simulink model "dbm_2020b"  (R2020b)
settings: Solver=FixedStepAuto  StartTime=0.0  StopTime=50  FixedStep=0.01  RelTol=1e-3
libraries: simulink x1
settings Model: Creator=felix  LastModifiedBy=felix
settings OptimizationCC: DefaultParameterBehavior=Inlined  UseDivisionForNetSlopeComputation=on  GainParamInheritBuiltInType=on  UseFloatMulNetSlope=on  InlineInvariantSignals=on  EfficientFloat2IntCast=on  LifeSpan=1
settings DebuggingCC: SFMachineParentedDataDiag=error
settings HardwareCC: ProdLongLongMode=on
settings SFSimCC: MATLABDynamicMemAlloc=off
settings RTWCC: GenerateReport=on  LaunchReport=on
settings CodeAppCC: ForceParamTrailComments=on
settings GRTTargetCC: CombineSignalStateStructs=on  MatFileLogging=off  SupportVariableSizeSignals=on

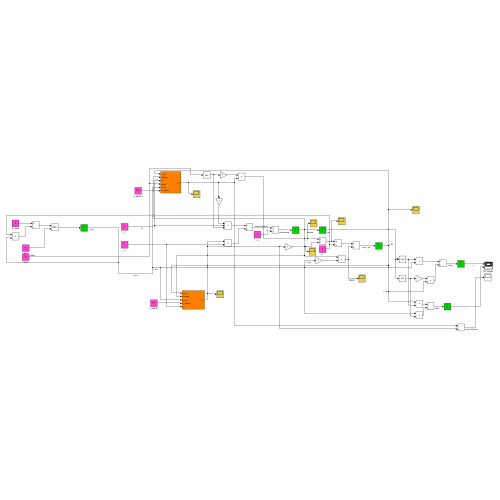
[thumbnail: Simulink's stored preview of the top-level diagram]
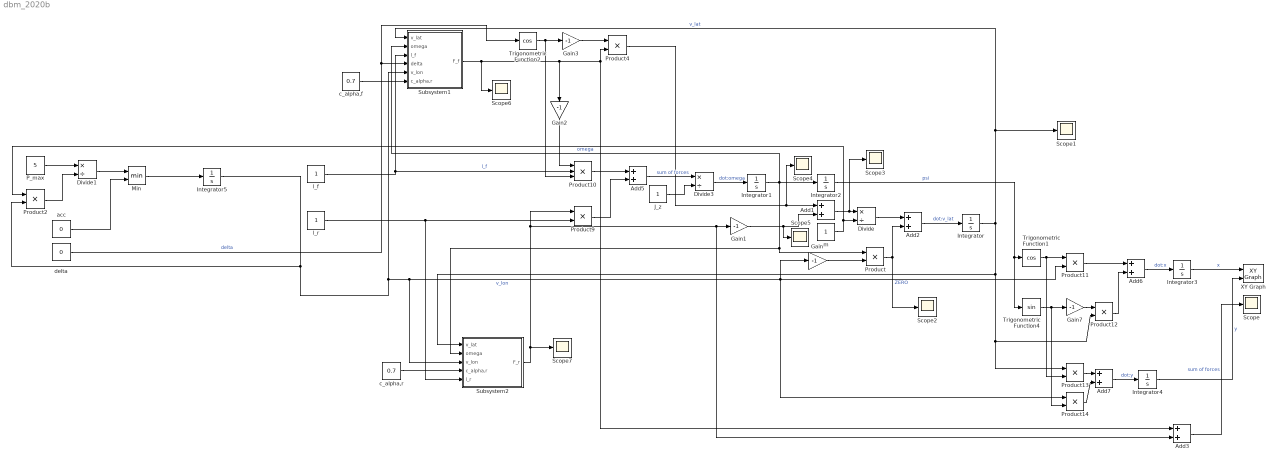
== system dbm_2020b ==
  Add{1..3,5..7} (6 alike) : Sum
  Divide : Product  Inputs=*/
  Divide1 : Product  Inputs=*/
  Divide3 : Product  Inputs=*/
  Gain{,1..3,7} (5 alike) : Gain  Gain=-1
  Integrator{,1..4} (5 alike) : Integrator
  Integrator5 : Integrator  InitialCondition=1
  J_z : Constant
  Min : MinMax  Inputs=2
  P_max : Constant  Value=5
  Product{,2,4,9,11..14} (8 alike) : Product
  Product10 : Product  Inputs=3
  Scope{,1..7} (8 alike) : Scope
  Subsystem1 : Subsystem
  Subsystem2 : Subsystem
  Trigonometric Function1 : Trigonometry  Operator=cos
  Trigonometric Function2 : Trigonometry  Operator=cos
  Trigonometric Function4 : Trigonometry
  XY Graph : simulink/Sinks/XY Graph  xmin=-1  xmax=1  ymin=-1  ymax=1  st=-1
  acc : Constant  Value=0
  c_alpha,f : Constant  Value=0.7
  c_alpha,r : Constant  Value=0.7
  delta : Constant  Value=0
  l_f : Constant
  l_r : Constant
  m : Constant
  wires:
  m/1 -> Divide/2, Product2/1
  Divide/1 -> Add2/1
  Integrator/1 -> Subsystem2/1(v_lat), Product13/1, Product12/2, Subsystem1/1(v_lat), Scope1/1  "v_lat"
  Integrator1/1 -> Subsystem1/2(omega), Integrator2/1, Product/1, Subsystem2/2(omega)  "omega"
  Integrator5/1 -> Subsystem2/3(v_lon), Product14/1, Product11/2, Gain/1, Subsystem1/5(v_lon), Product2/2  "v_lon"
  Gain/1 -> Product/2
  l_r/1 -> Subsystem2/5(l_r), Product9/2
  Product/1 -> Add2/2, Scope2/1  "ZERO"
  delta/1 -> Trigonometric Function2/1, Subsystem1/4(delta)  "delta"
  Trigonometric Function2/1 -> Product10/3, Gain3/1
  Gain3/1 -> Product4/1
  l_f/1 -> Product10/2, Subsystem1/3(l_f)  "l_f"
  Add1/1 -> Scope3/1, Divide/1
  J_z/1 -> Divide3/2
  Product10/1 -> Add5/1
  Product9/1 -> Add5/2
  Add5/1 -> Divide3/1  "sum of forces"
  Divide3/1 -> Integrator1/1  "dot:omega"
  Integrator2/1 -> Trigonometric Function4/1, Trigonometric Function1/1  "psi"
  Integrator3/1 -> XY Graph/1  "x"
  Trigonometric Function1/1 -> Product11/1, Product13/2
  Product11/1 -> Add6/1
  Trigonometric Function4/1 -> Product14/2, Gain7/1
  Product12/1 -> Add6/2
  Add6/1 -> Integrator3/1  "dot:x"
  Integrator4/1 -> XY Graph/2  "y"
  Product13/1 -> Add7/1
  Add7/1 -> Integrator4/1  "dot:y"
  Product14/1 -> Add7/2
  Gain7/1 -> Product12/1
  Product4/1 -> Scope4/1, Add1/1
  Subsystem2/1(F_r) -> Scope7/1, Add3/2, Gain1/1, Product9/1
  c_alpha,r/1 -> Subsystem2/4(c_alpha,r)
  Subsystem1/1(F_f) -> Scope6/1, Add3/1, Product4/2, Gain2/1
  c_alpha,f/1 -> Subsystem1/6(c_alpha,r)
  Gain1/1 -> Scope5/1, Add1/2
  Add2/1 -> Integrator/1  "dot:v_lat"
  Gain2/1 -> Product10/1
  P_max/1 -> Divide1/1
  Product2/1 -> Divide1/2
  Divide1/1 -> Min/1
  acc/1 -> Min/2
  Min/1 -> Integrator5/1
  Add3/1 -> Scope/1  "sum of forces"

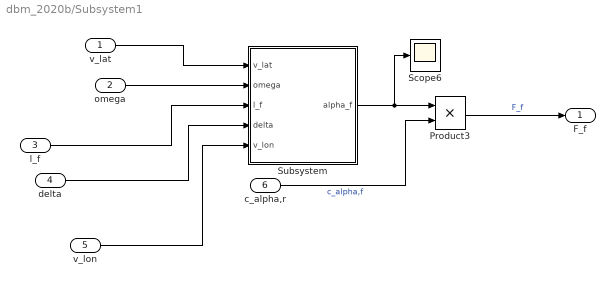
== system dbm_2020b/Subsystem1 ==
  v_lat : Inport
  omega : Inport  Port=2
  l_f : Inport  Port=3
  delta : Inport  Port=4
  v_lon : Inport  Port=5
  c_alpha,r : Inport  Port=6
  Product3 : Product
  Scope6 : Scope
  Subsystem : Subsystem
  F_f : Outport
  wires:
  Subsystem/1(alpha_f) -> Scope6/1, Product3/1
  v_lat/1 -> Subsystem/1(v_lat)
  Product3/1 -> F_f/1  "F_f"
  v_lon/1 -> Subsystem/5(v_lon)
  omega/1 -> Subsystem/2(omega)
  l_f/1 -> Subsystem/3(l_f)
  delta/1 -> Subsystem/4(delta)
  c_alpha,r/1 -> Product3/2  "c_alpha,f"

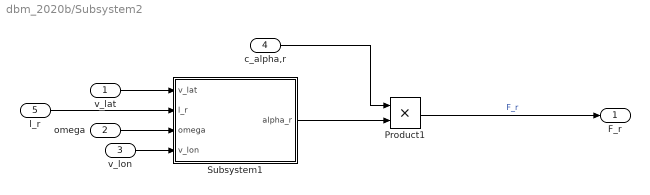
== system dbm_2020b/Subsystem2 ==
  v_lat : Inport
  omega : Inport  Port=2
  v_lon : Inport  Port=3
  c_alpha,r : Inport  Port=4
  l_r : Inport  Port=5
  Product1 : Product
  Subsystem1 : Subsystem
  F_r : Outport
  wires:
  v_lat/1 -> Subsystem1/1(v_lat)
  c_alpha,r/1 -> Product1/1
  Subsystem1/1(alpha_r) -> Product1/2
  l_r/1 -> Subsystem1/2(l_r)
  omega/1 -> Subsystem1/3(omega)
  Product1/1 -> F_r/1  "F_r"
  v_lon/1 -> Subsystem1/4(v_lon)

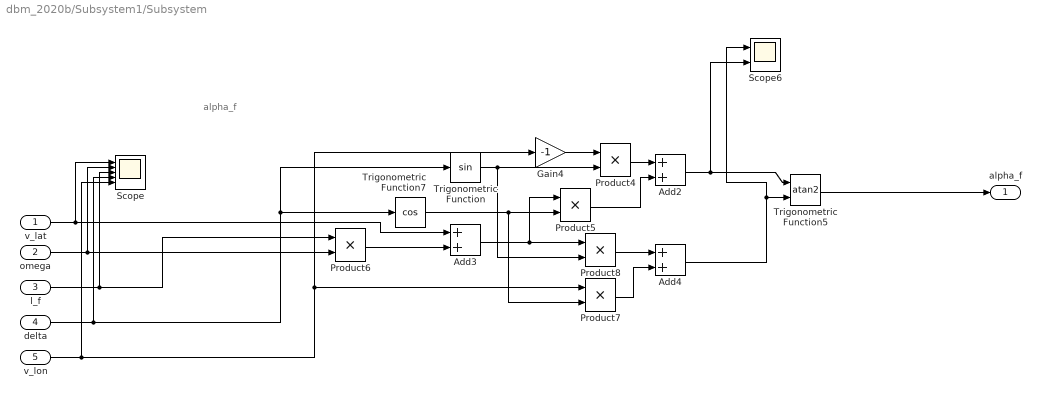
== system dbm_2020b/Subsystem1/Subsystem ==
  note: alpha_f
  v_lat : Inport
  omega : Inport  Port=2
  l_f : Inport  Port=3
  delta : Inport  Port=4
  v_lon : Inport  Port=5
  Add2 : Sum
  Add3 : Sum
  Add4 : Sum
  Gain4 : Gain  Gain=-1
  Product{4..8} (5 alike) : Product
  Scope : Scope  NumInputPorts=5
  Scope6 : Scope  NumInputPorts=2
  Trigonometric Function : Trigonometry
  Trigonometric Function5 : Trigonometry  Operator=atan2
  Trigonometric Function7 : Trigonometry  Operator=cos
  alpha_f : Outport
  wires:
  v_lon/1 -> Product7/1, Gain4/1, Scope/5
  Add2/1 -> Trigonometric Function5/1, Scope6/2
  Add4/1 -> Scope6/1, Trigonometric Function5/2
  Product5/1 -> Add2/2
  Trigonometric Function/1 -> Product8/2, Product4/2
  Product4/1 -> Add2/1
  Gain4/1 -> Product4/1
  Product6/1 -> Add3/2
  Add3/1 -> Product8/1, Product5/1
  delta/1 -> Trigonometric Function7/1, Trigonometric Function/1, Scope/4
  Product7/1 -> Add4/2
  v_lat/1 -> Scope/1, Add3/1
  Trigonometric Function7/1 -> Product7/2, Product5/2
  Product8/1 -> Add4/1
  l_f/1 -> Scope/3, Product6/1
  Trigonometric Function5/1 -> alpha_f/1
  omega/1 -> Scope/2, Product6/2

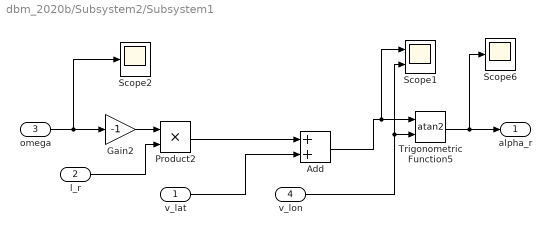
== system dbm_2020b/Subsystem2/Subsystem1 ==
  v_lat : Inport
  l_r : Inport  Port=2
  omega : Inport  Port=3
  v_lon : Inport  Port=4
  Add : Sum
  Gain2 : Gain  Gain=-1
  Product2 : Product
  Scope1 : Scope  NumInputPorts=2
  Scope2 : Scope
  Scope6 : Scope
  Trigonometric Function5 : Trigonometry  Operator=atan2
  alpha_r : Outport
  wires:
  Add/1 -> Scope1/1, Trigonometric Function5/1
  l_r/1 -> Product2/2
  omega/1 -> Scope2/1, Gain2/1
  Gain2/1 -> Product2/1
  v_lon/1 -> Scope1/2, Trigonometric Function5/2
  Product2/1 -> Add/1
  v_lat/1 -> Add/2
  Trigonometric Function5/1 -> Scope6/1, alpha_r/1
